simulink model "Demo_AUV_VA"  (R2014a)
settings: Solver=FixedStepDiscrete  StartTime=0.0  StopTime=inf  FixedStep=0.01  RelTol=1e-3
undefined symbols (not defined in the file or in its folder): clock, lib_affectiveChar_behavior, notImitateSmile, Stateflow
libraries: simulink x6, realtime_pacer_lib x2
(part 1 of 2)
settings Model: Creator=root180  LastModifiedBy=root180

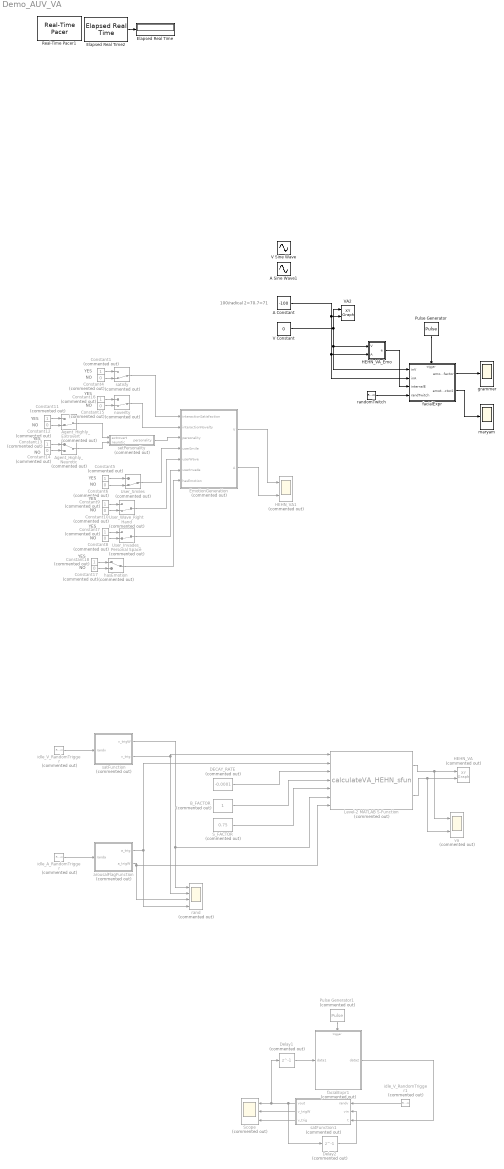
== system Demo_AUV_VA ==
  note: 100/radical 2=70.7=71
  note: NO
  note: NO
  note: YES
  note: YES
  note: NO
  note: YES
  note: NO
  note: NO
  note: NO
  note: NO
  note: NO
  note: YES
  note: YES
  note: YES
  note: YES
  note: YES
  A Constant : Constant  Value=-100
  A Sine Wave1 : Sin  Amplitude=100  Frequency=0.1  SampleTime=0.01
  Agent_Highly_Extrovert : ManualSwitch  Commented=on  CurrentSetting=0
  Agent_Highly_Neurotic : ManualSwitch  Commented=on
  B_FACTOR : Constant  Commented=on
  Constant{1,5,7,9,16,18} (6 alike) : Constant  Commented=on  OutDataTypeStr=double
  Constant{4,6,8,10,15,17} (6 alike) : Constant  Commented=on  Value=0  OutDataTypeStr=double
  Constant11 : Constant  Commented=on  OutDataTypeStr=boolean
  Constant12 : Constant  Commented=on  Value=0  OutDataTypeStr=boolean
  Constant13 : Constant  Commented=on  OutDataTypeStr=boolean
  Constant14 : Constant  Commented=on  Value=0  OutDataTypeStr=boolean
  DECAY_RATE : Constant  Commented=on  Value=-0.0001
  Delay1 : Delay  Commented=on  DelayLength=1  InitialCondition=0  SampleTime=0.01
  Delay2 : Delay  Commented=on  DelayLength=1  InitialCondition=0  SampleTime=0.01
  Elapsed Real Time : Display
      settings: Decimation=2
  Elapsed Real Time2 : realtime_pacer_lib/Elapsed Real Time
  EmotionGeneration : Subsystem  Commented=on
  HEHN_VA : simulink/Sinks/XY Graph  Commented=on  xmin=-110  xmax=100  ymin=-110  ymax=110  st=-1
  HEHN_VA1 : Scope  Commented=on  NumInputPorts=2
      settings: YMin=-0.65~21.8  YMax=0.3~23.9  SaveName=ScopeData4
  HEHN_VA_Emo : Truth Table  TreatAsAtomicUnit=on
  Level-2 MATLAB S-Function : M-S-Function  Commented=on  FunctionName=calculateVA_HEHN_sfun
  Pulse Generator : DiscretePulseGenerator  SampleTime=0.01
  Pulse Generator1 : DiscretePulseGenerator  Commented=on  Period=20  PulseWidth=10  SampleTime=0.01
  Real-Time Pacer1 : realtime_pacer_lib/Real-Time Pacer  simTimePerRealTime=1
  S_FACTOR : Constant  Commented=on  Value=0.75
  Scope : Scope  Commented=on  NumInputPorts=3
      settings: YMin=0.57~0.285~0.95  YMax=0.63~0.315~1.05  SaveName=ScopeData7
  User_Invades_Personal Space : ManualSwitch  Commented=on  CurrentSetting=0
  User_Smiles : ManualSwitch  Commented=on  CurrentSetting=0
  User_Wave_Right Hand : ManualSwitch  Commented=on  CurrentSetting=0
  V Constant : Constant  Value=0
  V Sine Wave : Sin  Amplitude=100  SampleTime=0.01
  VA2 : simulink/Sinks/XY Graph  xmin=-110  xmax=100  ymin=-110  ymax=110  st=-1
  arousalFlagFunction : MATLAB Function  Commented=on  TreatAsAtomicUnit=on
  facialExpr : Stateflow chart  TreatAsAtomicUnit=on
  facialExpr1 : Stateflow chart  Commented=on  TreatAsAtomicUnit=on
  grammer : Scope
  hasEmotion : ManualSwitch  Commented=on
  idle_A_RandomTrigger : UniformRandomNumber  Commented=on  Minimum=0  Maximum=100.9999  Seed=sum(10*clock)  SampleTime=0.1
  idle_V_RandomTrigger : UniformRandomNumber  Commented=on  Minimum=0  Maximum=100.9999  Seed=sum(10*clock)  SampleTime=0.1
  idle_V_RandomTrigger1 : UniformRandomNumber  Commented=on  Minimum=0  Maximum=100.9999  Seed=sum(10*clock)  SampleTime=0.01
  maryam : Scope
      settings: SaveName=ScopeData8
  noverlty : ManualSwitch  Commented=on  CurrentSetting=0
  rand : Scope  Commented=on  NumInputPorts=4
      settings: TickLabels=on  YMin=0~-1~-90~-5  YMax=1~1~-20~5  SaveName=ScopeData2  MaxDataPoints=100000
  randomTwitch : UniformRandomNumber  Minimum=0  Maximum=100.9999  Seed=sum(10*clock)  SampleTime=0.01
  satFunction : MATLAB Function  Commented=on  TreatAsAtomicUnit=on
  satFunction1 : MATLAB Function  Commented=on  TreatAsAtomicUnit=on
  satisfy : ManualSwitch  Commented=on  CurrentSetting=0
  setPersonality : MATLAB Function  Commented=on  TreatAsAtomicUnit=on
  va : Scope  Commented=on  NumInputPorts=2
      settings: YMin=-5~-5  YMax=5~5  SaveName=ScopeData3
  wires:
  Pulse Generator/1 -> facialExpr/Trigger
  facialExpr/1(emotion_amount_factor) -> grammer/1
  V Constant/1 -> VA2/1, HEHN_VA_Emo/1(V), facialExpr/1(inV)
  A Constant/1 -> facialExpr/2(inA), HEHN_VA_Emo/2(A), VA2/2
  EmotionGeneration/1(V) -> HEHN_VA1/1
  EmotionGeneration/2(A) -> HEHN_VA1/2
  User_Invades_Personal Space/1 -> EmotionGeneration/6(userInvade)
  User_Smiles/1 -> EmotionGeneration/4(userSmile)
  setPersonality/1(personality) -> EmotionGeneration/3(personality)
  hasEmotion/1 -> EmotionGeneration/7(hasEmotion)
  Constant9/1 -> User_Wave_Right Hand/1
  Constant11/1 -> Agent_Highly_Extrovert/1
  Constant13/1 -> Agent_Highly_Neurotic/1
  Constant1/1 -> satisfy/1
  Constant6/1 -> User_Smiles/2
  Constant12/1 -> Agent_Highly_Extrovert/2
  Constant18/1 -> hasEmotion/1
  Constant8/1 -> User_Invades_Personal Space/2
  Agent_Highly_Neurotic/1 -> setPersonality/2(neurotic)
  Constant15/1 -> noverlty/2
  Constant17/1 -> hasEmotion/2
  Constant7/1 -> User_Invades_Personal Space/1
  Constant4/1 -> satisfy/2
  Constant10/1 -> User_Wave_Right Hand/2
  noverlty/1 -> EmotionGeneration/2(interactionNovelty)
  Constant16/1 -> noverlty/1
  Constant5/1 -> User_Smiles/1
  User_Wave_Right Hand/1 -> EmotionGeneration/5(userWave)
  Agent_Highly_Extrovert/1 -> setPersonality/1(extrovert)
  satisfy/1 -> EmotionGeneration/1(interactionSatisfaction)
  Constant14/1 -> Agent_Highly_Neurotic/2
  idle_V_RandomTrigger/1 -> satFunction/1(randv)
  B_FACTOR/1 -> Level-2 MATLAB S-Function/4
  DECAY_RATE/1 -> Level-2 MATLAB S-Function/3
  idle_A_RandomTrigger/1 -> arousalFlagFunction/1(randa)
  S_FACTOR/1 -> Level-2 MATLAB S-Function/5
  Level-2 MATLAB S-Function/2 -> va/2, HEHN_VA/2
  Level-2 MATLAB S-Function/1 -> va/1, HEHN_VA/1
  satFunction/2(v_trig) -> rand/2, Level-2 MATLAB S-Function/1
  arousalFlagFunction/1(a_trig) -> rand/4, Level-2 MATLAB S-Function/2
  arousalFlagFunction/2(a_trigW) -> Level-2 MATLAB S-Function/7, rand/3
  satFunction/1(v_trigW) -> Level-2 MATLAB S-Function/6, rand/1
  Elapsed Real Time2/1 -> Elapsed Real Time/1
  idle_V_RandomTrigger1/1 -> satFunction1/1(randv)
  satFunction1/1(vout) -> Delay2/1, Scope/1, Delay1/1
  satFunction1/3(v_trig) -> Scope/3
  satFunction1/2(v_trigW) -> Scope/2
  Pulse Generator1/1 -> facialExpr1/Trigger
  Delay1/1 -> facialExpr1/1(data1)
  facialExpr1/1(data2) -> satFunction1/3(t)
  Delay2/1 -> satFunction1/2(vin)
  HEHN_VA_Emo/1(e) -> facialExpr/3(internalE)
  facialExpr/2(emotion_amount_factor2) -> maryam/1
  randomTwitch/1 -> facialExpr/4(randTwitch)

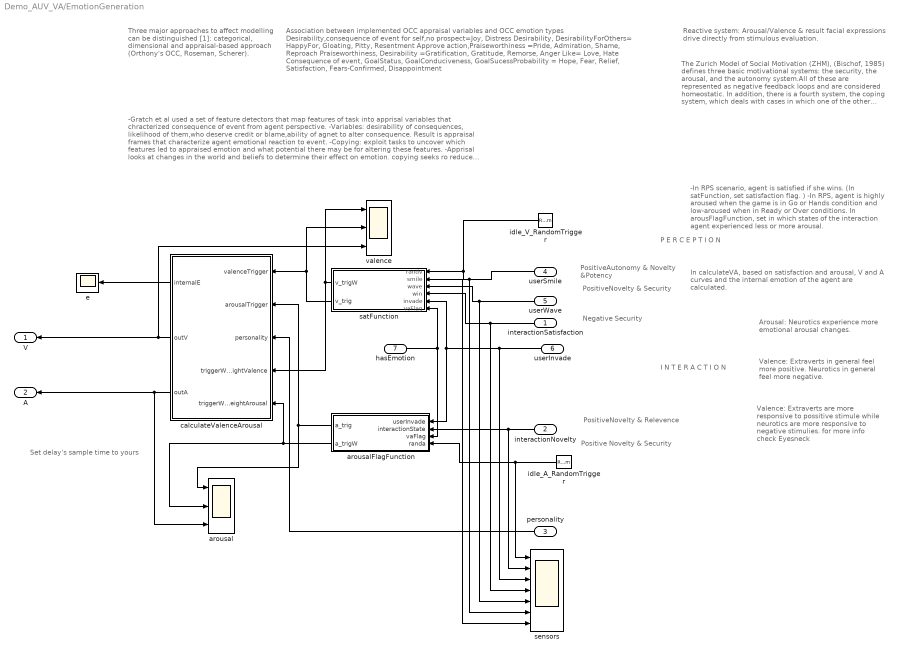
== system Demo_AUV_VA/EmotionGeneration ==
  note: P
      | E
      | R
      | C
      | E
      | P
      | T
      | I
      | O
      | N
  note: PositiveNovelty &
      | Relevence
  note: The Zurich Model of Social Motivation (ZHM), (Bischof, 1985) defines three basic motivational systems: the security, the arousal, and the autonomy system.All of these are represented as negative feedback loops and are considered homeostatic. In addition, there is a fourth system, the coping system, which deals with cases in which one of the other systems gets blocked and cannot operate in its usual manner.( Bernardet and Schneider, 2013)
  note: PositiveNovelty &
      | Security
  note: Three major approaches to affect modelling can be distinguished [1]: categorical, dimensional and appraisal-based approach (Orthony's OCC, Roseman, Scherer).
  note: Reactive system: Arousal/Valence & result facial expressions drive directly from stimulous evaluation.
  note: Association between implemented OCC appraisal variables and OCC emotion types
      | Desirability,consequence of event for self,no prospect=Joy, Distress
      | Desirability, DesirabilityForOthers= HappyFor, Gloating, Pitty, Resentment
      | Approve action,Praiseworthiness =Pride, Admiration, Shame, Reproach
      | Praiseworthiness, Desirability =Gratification, Gratitude, Remorse, Anger
      | Like= Love, Hate
      | Consequence of event, GoalStatus, GoalConduciveness, GoalSucessProbability = Hope, Fear, Relief, Satisfaction, Fears-Confirmed, Disappointment
  note: -Gratch et al used a set of feature detectors that map features of task into apprisal variables that chracterized consequence of event from agent perspective.
      | -Variables: desirability of consequences, likelihood of them,who deserve credit or blame,ability of agnet to alter consequence. Result is appraisal frames that characterize agent emotional reaction to event.
      | -Copying: exploit tasks to uncover which features led to appraised emotion and what potential there may be for altering these features.
      | -Apprisal looks at changes in the world and beliefs to determine their effect on emotion.
      | copying seeks ro reduce (-) emotions by making changes to world or beliefs (problem-focused v.s. emotion-focused)
      | -For more info check Toward Virtual Humans, Swartout,w., et al (2006)
  note: In calculateVA, based on satisfaction and arousal, V and A curves and the internal emotion of the agent are calculated.
  note: Set delay's sample time to yours
  note: -In RPS scenario, agent is satisfied if she wins. (In satFunction, set satisfaction flag. )
      | -In RPS, agent is highly aroused when the game is in Go or Hands condition and low-aroused when in Ready or Over conditions.
      | In arousFlagFunction, set in which states of the interaction agent experienced less or more arousal.
  note: Valence: Extraverts are more responsive to possitive stimule while neurotics are more responsive to negative stimulies. for more info check Eyesneck
  note: Valence: Extraverts in general feel more positive. Neurotics in general feel more negative.
  note: Arousal: Neurotics experience more emotional arousal changes.
  note: Positive Novelty &
      | Security
  note: Negative Security
  note: PositiveAutonomy &
      | Novelty &Potency
  note: I
      | N
      | T
      | E
      | R
      | A
      | C
      | T
      | I
      | O
      | N
  interactionSatisfaction : Inport
  interactionNovelty : Inport  Port=2
  personality : Inport  Port=3
  userSmile : Inport  Port=4
  userWave : Inport  Port=5
  userInvade : Inport  Port=6
  hasEmotion : Inport  Port=7
  arousal : Scope  NumInputPorts=3
      settings: TickLabels=on  YMin=-1~0~0  YMax=1~0.1~90  SaveName=ScopeData12  MaxDataPoints=200000
  arousalFlagFunction : MATLAB Function  TreatAsAtomicUnit=on
  calculateValenceArousal : Subsystem
  e : Scope
      settings: TickLabels=on  YMin=0  YMax=1  MaxDataPoints=100000
  idle_A_RandomTrigger : UniformRandomNumber  Minimum=0  Maximum=100.9999  Seed=sum(10*clock)  SampleTime=0.01
  idle_V_RandomTrigger : UniformRandomNumber  Minimum=0  Maximum=100.9999  Seed=sum(10*clock)  SampleTime=0.01
  satFunction : MATLAB Function  TreatAsAtomicUnit=on
  sensors : Scope  NumInputPorts=7
      settings: YMin=0.95~-20.15~-20.15~-5~-5~-5~-5  YMax=1.05~-19.15~-19.15~5~5~5~5  SaveName=ScopeData10  MaxDataPoints=20000
  valence : Scope  NumInputPorts=3
      settings: TickLabels=on  YMin=0~-1~-90  YMax=1~1~-20  SaveName=ScopeData14  MaxDataPoints=100000
  V : Outport
  A : Outport  Port=2
  wires:
  arousalFlagFunction/1(a_trig) -> calculateValenceArousal/2(arousalTrigger), arousal/1
  calculateValenceArousal/2(outV) -> V/1, valence/3
  calculateValenceArousal/3(outA) -> A/1, arousal/3
  personality/1 -> calculateValenceArousal/3(personality)
  interactionNovelty/1 -> sensors/2, arousalFlagFunction/2(interactionState)
  interactionSatisfaction/1 -> sensors/4, satFunction/4(win)
  userInvade/1 -> sensors/3, arousalFlagFunction/1(userInvade), satFunction/5(invade)
  userWave/1 -> sensors/5, satFunction/3(wave)
  satFunction/1(v_trigW) -> valence/1, calculateValenceArousal/4(triggerWeightValence)
  arousalFlagFunction/2(a_trigW) -> arousal/2, calculateValenceArousal/5(triggerWeightArousal)
  hasEmotion/1 -> satFunction/6(vaFlag), arousalFlagFunction/3(vaFlag)
  idle_V_RandomTrigger/1 -> sensors/7, satFunction/1(randv)
  idle_A_RandomTrigger/1 -> sensors/1, arousalFlagFunction/4(randa)
  satFunction/2(v_trig) -> calculateValenceArousal/1(valenceTrigger), valence/2
  calculateValenceArousal/1(internalE) -> e/1
  userSmile/1 -> satFunction/2(smile), sensors/6

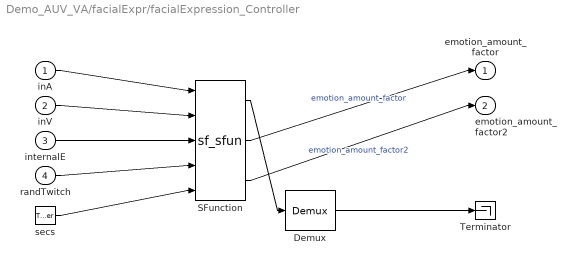
== system Demo_AUV_VA/facialExpr/facialExpression_Controller ==
  inA : Inport
  inV : Inport  Port=2
  internalE : Inport  Port=3
  randTwitch : Inport  Port=4
  secs : TriggerPort  ShowOutputPort=on
  " Demux " : Demux  Outputs=1
  " SFunction " : S-Function  Tag=Stateflow S-Function Demo_AUV_VA 50  FunctionName=sf_sfun  PortCounts=[5 3]  EnableBusSupport=off
  " Terminator " : Terminator
  emotion_amount_factor : Outport
  emotion_amount_factor2 : Outport  Port=2
  wires:
  inA/1 -> " SFunction "/1
  inV/1 -> " SFunction "/2
  internalE/1 -> " SFunction "/3
  randTwitch/1 -> " SFunction "/4
  " SFunction "/2 -> emotion_amount_factor/1  "emotion_amount_factor"
  " SFunction "/3 -> emotion_amount_factor2/1  "emotion_amount_factor2"
  " Demux "/1 -> " Terminator "/1
  secs/1 -> " SFunction "/5
  " SFunction "/1 -> " Demux "/1

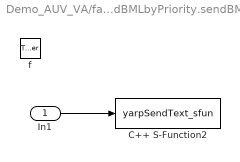
== system Demo_AUV_VA/facialExpr/sendBMLbyPriority.sendBML ==
  In1 : Inport  OutDataTypeStr=double  PortDimensions=[2000 1]
  f : TriggerPort  TriggerType=function-call
      settings: CopyFcn=Stateflow.SLINSF.SimulinkMan.removeBlockPreDeleteFcn  PreDeleteFcn=Stateflow.SLINSF.SimulinkMan.unsafePredeleteFcn
  C++ S-Function2 : S-Function  FunctionName=yarpSendText_sfun  Parameters='/sim/out/bml0', '/SB/in/bml'  EnableBusSupport=off
  wires:
  In1/1 -> C++ S-Function2/1

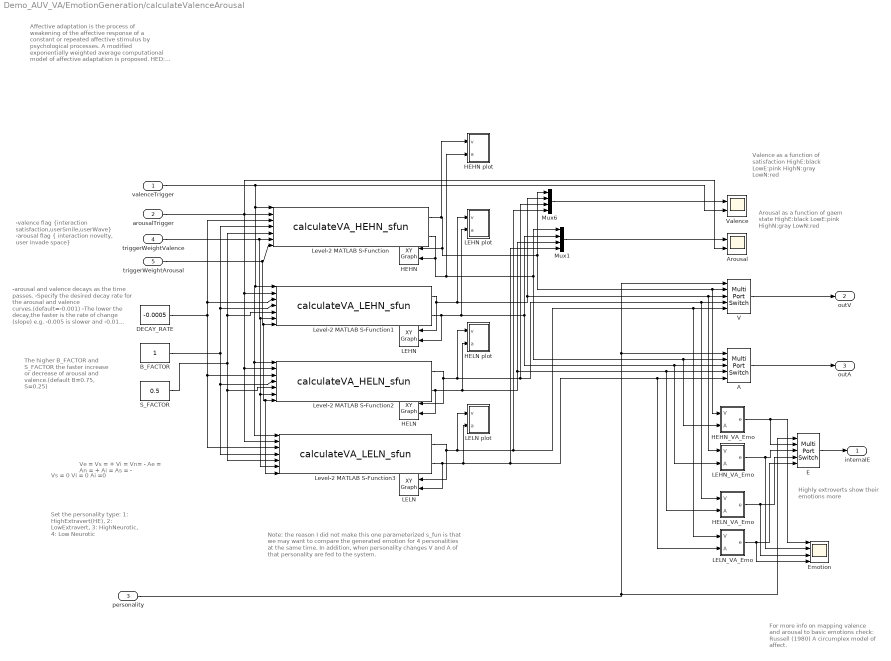
== system Demo_AUV_VA/EmotionGeneration/calculateValenceArousal ==
  note: Highly extroverts show their emotions more
  note: Note: the reason I did not make this one parameterized s_fun is that we may want to compare the generated emotion for 4 personalities at the same time.
      | In addition, when personality changes V and A of that personality are fed to the system.
  note: For more info on mapping valence and arousal to basic emotions check: Russell (1980) A circumplex model of affect.
  note: Valence as a  function of satisfaction
      | HighE:black
      | LowE:pink
      | HighN:gray
      | LowN:red
  note: Set the personality type:
      | 1: HighExtravert(HE),
      | 2: LowExtravert,
      | 3: HighNeurotic,
      | 4: Low Neurotic
  note: The higher B_FACTOR and S_FACTOR the faster increase or decrease of arousal and valence.(default B=0.75, S=0.25)
  note: -arousal and valence decays as the time passes.
      | -Specify the desired decay rate for the arousal and valence curves.(default=-0.001)
      | -The lower the decay,the faster is the rate of change (slope)
      | e.g. -0.005 is slower and -0.01 faster
  note: Vs = 0
      | Vi = 0
      | Ai =0
  note: Ve = Vs = +
      | Vi = Vn= -
      | Ae = An = +
      | Ai = As  = -
  note: Arousal as a function of gaem state
      | HighE:black
      | LowE:pink
      | HighN:gray
      | LowN:red
  note: Affective adaptation is the process of weakening of the affective response of a constant or repeated affective stimulus by psychological processes. A modified exponentially weighted average computational model of affective adaptation is proposed.
      |
      | HED: A Computational Model of Affective Adaptation and Emotion Dynamics, John E. Steephen
  note: -valence flag {interaction satisfaction,userSmile,userWave}
      | -arousal flag { interaction novelty, user invade space}
  valenceTrigger : Inport  OutDataTypeStr=double  PortDimensions=1
  arousalTrigger : Inport  Port=2  OutDataTypeStr=double  PortDimensions=1
  personality : Inport  Port=3  OutDataTypeStr=double  PortDimensions=1
  triggerWeightValence : Inport  Port=4  OutDataTypeStr=double  PortDimensions=1
  triggerWeightArousal : Inport  Port=5  OutDataTypeStr=double  PortDimensions=1
  A : MultiPortSwitch  Inputs=4
  Arousal : Scope  NumInputPorts=2
      settings: YMin=-6~-1  YMax=5~1  SaveName=ScopeData11  MaxDataPoints=20000
  B_FACTOR : Constant
  DECAY_RATE : Constant  Value=-0.0005
  E : MultiPortSwitch  Inputs=4
  Emotion : Scope  NumInputPorts=4
      settings: TimeRange=50  YMin=6.65~5.7~5.7~5.7  YMax=7.35~6.3~6.3~6.3  SaveName=ScopeData5  MaxDataPoints=10000
  HEHN : simulink/Sinks/XY Graph  xmin=-110  xmax=100  ymin=-110  ymax=110  st=-1
  HEHN plot : MATLAB Function  TreatAsAtomicUnit=on
  HEHN_VA_Emo : Truth Table  TreatAsAtomicUnit=on
  HELN : simulink/Sinks/XY Graph  xmin=-110  xmax=110  ymin=-110  ymax=110  st=-1
  HELN plot : MATLAB Function  TreatAsAtomicUnit=on
  HELN_VA_Emo : Truth Table  TreatAsAtomicUnit=on
  LEHN : simulink/Sinks/XY Graph  xmin=-110  xmax=110  ymin=-110  ymax=110  st=-1
  LEHN plot : MATLAB Function  TreatAsAtomicUnit=on
  LEHN_VA_Emo : Truth Table  TreatAsAtomicUnit=on
  LELN : simulink/Sinks/XY Graph  xmin=-110  xmax=110  ymin=-110  ymax=110  st=-1
  LELN plot : MATLAB Function  TreatAsAtomicUnit=on
  LELN_VA_Emo : Truth Table  TreatAsAtomicUnit=on
  Level-2 MATLAB S-Function : M-S-Function  FunctionName=calculateVA_HEHN_sfun
  Level-2 MATLAB S-Function1 : M-S-Function  FunctionName=calculateVA_LEHN_sfun
  Level-2 MATLAB S-Function2 : M-S-Function  FunctionName=calculateVA_HELN_sfun
  Level-2 MATLAB S-Function3 : M-S-Function  FunctionName=calculateVA_LELN_sfun
  Mux1 : Mux
  Mux6 : Mux
  S_FACTOR : Constant  Value=0.5
  V : MultiPortSwitch  Inputs=4
  Valence : Scope  NumInputPorts=2
      settings: TimeRange=10  YMin=-12~-1  YMax=10~1  SaveName=ScopeData6  MaxDataPoints=20000
  internalE : Outport
  outV : Outport  Port=2
  outA : Outport  Port=3
  wires:
  valenceTrigger/1 -> Valence/2, Level-2 MATLAB S-Function/1, Level-2 MATLAB S-Function3/1, Level-2 MATLAB S-Function2/1, Level-2 MATLAB S-Function1/1
  Level-2 MATLAB S-Function/2 -> HEHN/2, HEHN plot/2(a), HEHN_VA_Emo/2(A), A/2, Mux1/1
  arousalTrigger/1 -> Arousal/2, Level-2 MATLAB S-Function/2, Level-2 MATLAB S-Function3/2, Level-2 MATLAB S-Function2/2, Level-2 MATLAB S-Function1/2
  Level-2 MATLAB S-Function1/2 -> LEHN plot/2(a), LEHN_VA_Emo/2(A), A/3, Mux1/2, LEHN/2
  Level-2 MATLAB S-Function/1 -> HEHN plot/1(v), Mux6/1, HEHN_VA_Emo/1(V), V/2, HEHN/1
  Level-2 MATLAB S-Function1/1 -> LEHN plot/1(v), Mux6/2, LEHN_VA_Emo/1(V), V/3, LEHN/1
  Level-2 MATLAB S-Function2/2 -> HELN plot/2(a), Mux1/3, HELN_VA_Emo/2(A), A/4, HELN/2
  Level-2 MATLAB S-Function3/2 -> LELN plot/2(a), LELN_VA_Emo/2(A), A/5, Mux1/4, LELN/2
  Level-2 MATLAB S-Function2/1 -> HELN plot/1(v), HELN_VA_Emo/1(V), V/4, Mux6/3, HELN/1
  Level-2 MATLAB S-Function3/1 -> LELN plot/1(v), LELN_VA_Emo/1(V), V/5, Mux6/4, LELN/1
  Mux1/1 -> Arousal/1
  Mux6/1 -> Valence/1
  DECAY_RATE/1 -> Level-2 MATLAB S-Function/3, Level-2 MATLAB S-Function1/3, Level-2 MATLAB S-Function2/3, Level-2 MATLAB S-Function3/3
  B_FACTOR/1 -> Level-2 MATLAB S-Function/4, Level-2 MATLAB S-Function1/4, Level-2 MATLAB S-Function3/4, Level-2 MATLAB S-Function2/4
  S_FACTOR/1 -> Level-2 MATLAB S-Function3/5, Level-2 MATLAB S-Function2/5, Level-2 MATLAB S-Function1/5, Level-2 MATLAB S-Function/5
  V/1 -> outV/1
  A/1 -> outA/1
  personality/1 -> E/1, V/1, A/1
  triggerWeightValence/1 -> Level-2 MATLAB S-Function3/6, Level-2 MATLAB S-Function2/6, Level-2 MATLAB S-Function1/6, Level-2 MATLAB S-Function/6
  triggerWeightArousal/1 -> Level-2 MATLAB S-Function3/7, Level-2 MATLAB S-Function2/7, Level-2 MATLAB S-Function1/7, Level-2 MATLAB S-Function/7
  HEHN_VA_Emo/1(e) -> Emotion/1, E/2
  LEHN_VA_Emo/1(e) -> Emotion/2, E/3
  HELN_VA_Emo/1(e) -> Emotion/3, E/4
  LELN_VA_Emo/1(e) -> Emotion/4, E/5
  E/1 -> internalE/1

== matlab function Demo_AUV_VA/arousalFlagFunction ==
  data: a_trig output; a_trigW output; randa input
function [a_trig,a_trigW]= fcn(randa)
    a_trigW=0; 
    randTrigger=floor(randa);
    if(0<randTrigger)&&(randTrigger<30)
        a_trigW = a_trigW + 0.3;
    end
    if(30<randTrigger)&&(randTrigger<60)
        a_trigW = a_trigW - 0.3;
    end

    if(a_trigW>0)
        a_trig=1;
    elseif(a_trigW<0)
        a_trig=-1;
        a_trigW=abs(a_trigW);
    else
        a_trig=0;
    end

== matlab function Demo_AUV_VA/satFunction ==
  data: randv input; v_trigW output; v_trig output
function [v_trigW,v_trig]= fcn(randv)
    
    v_trigW=0;
    
    randTrigger=floor(randv);
    
    if(0<randTrigger)&&(randTrigger<30)
        v_trigW = v_trigW + 0.3;
    end
    if(30<randTrigger)&&(randTrigger<60)
        v_trigW = v_trigW - 0.3;
    end

    if(v_trigW>0)
        v_trig=1;
    elseif(v_trigW<0)
        v_trig=-1;
        v_trigW=abs(v_trigW);
    else
        v_trig=0;v_trigW=0;
    end

== stateflow chart Demo_AUV_VA/facialExpr ==
  state facialExpression_Controller [parallel]
    settings: executionOrder=1
  state sendBMLbyPriority [parallel]
    settings: executionOrder=2
    state sendH
      entry: BML=bmlsH(:,1);
      sendBML(BML);
      newBmlsH=removeQueue(bmlsH);
      bmlsH=newBmlsH;
    state init
      entry: n=encStr2Arr(' ');
      bmlsH=[n n n n n];
      bmlsM=[n n n n n];
      bmlsL=[n n n n n];
    state checkHighPriority
      entry:
      hEmpty=isEmptyQueue(bmlsH);
    state sendM
      entry: BML=bmlsM(:,1);
      sendBML(BML);
      newBmlsM= removeQueue(bmlsM);
      bmlsM=newBmlsM;
    state Mid
      entry:mEmpty=isEmptyQueue(bmlsM);
    state sendL
      entry: BML=bmlsL(:,1);
      sendBML(BML);
      newBmlsL= removeQueue(bmlsL);
      bmlsL=newBmlsL;
    state low
      entry:
      lEmpty=isEmptyQueue(bmlsL);
    note: Arrows' execution order is very importan here!
    state sendBML(In1) [function]
    sendH -> checkHighPriority
    checkHighPriority -> sendH [order 2] : [hEmpty~=1]
    (default) -> init
    init -> checkHighPriority
    checkHighPriority -> Mid [order 1] : [hEmpty==1]
    Mid -> checkHighPriority [order 4] : [mEmpty==1]
    sendM -> checkHighPriority [order 2]
    sendL -> checkHighPriority [order 3]
    low -> sendH [order 1] : [isEmptyQueue(bmlsH)~=1]
    Mid -> sendH [order 1] : [isEmptyQueue(bmlsH)~=1]
    sendM -> sendH [order 1] : [isEmptyQueue(bmlsH)~=1]
    sendL -> sendH [order 2] : [isEmptyQueue(bmlsH)~=1]
    Mid -> sendM [order 2] : [mEmpty~=1]
    Mid -> low [order 3] : [mEmpty==1]
    low -> Mid [order 4] : [lEmpty==1]
    low -> sendM [order 2] : [isEmptyQueue(bmlsM)~=1]
    sendL -> sendM [order 1] : [isEmptyQueue(bmlsM)~=1]
    low -> sendL [order 3] : [lEmpty~=1]
  data: In1 function_input double size=[2000 1]; bmls function_input; newBmls function_output; bmls function_input; empty function_output; inV input double size=1; inA input double size=1; bmlsL local double size=[2000,5]; newBmlsL local double size=[2000,5]; emotion_amount_factor output double size=[1,15]; hEmpty local double size=1; newBmlsM local double size=[2000,5]; bmlsM local double size=[2000,5]; newBmlsH local double size=[2000,5]; bmlsH local double size=[2000,5]; newBmlA local; BML local double size=[2000,1]; lEmpty local; mEmpty local; n local double size=[2000,1]; internalE input double size=1; emotion_amount_factor2 output double size=[1,6]; randTwitch input double size=1
  events: secs input RISING_EDGE_EVENT
  function newBmls=removeQueue(bmls):
    | function newBmls=removeQueue(bmls) 
    |     n=encStr2Arr(' ');
    |     newBmls=[n n n n n];
    |     newBmls(:,1)= bmls(:,2);
    |     newBmls(:,2)= bmls(:,3);
    |     newBmls(:,3)= bmls(:,4);
    |     newBmls(:,4)= bmls(:,5);
    |     newBmls(:,5)=encStr2Arr(' ');
  function empty=isEmptyQueue(bmls):
    | function empty=isEmptyQueue(bmls)
    | empty=1;
    | tempp=encStr2Arr(' ');
    | for i = 1:5
    |     if (isequal(bmls(:,i),tempp)==0)%there is a cell which is not equal to null
    |         empty=0;
    |         break
    |     end
    | end

== matlab function Demo_AUV_VA/satFunction1 ==
  data: vout output; randv input; v_trigW output; v_trig output; vin input; t input
function [vout,v_trigW,v_trig]= fcn(randv,vin,t)
%#codegen
    v_trigW=0;vout=0;
    randTrigger=floor(randv);
    if(0<randTrigger)&&(randTrigger<30)
        v_trigW = v_trigW + 0.3;
    end
    if(30<randTrigger)&&(randTrigger<60)
        v_trigW = v_trigW - 0.3;
    end
    if(v_trigW>0)
        v_trig=1;
    elseif(v_trigW<0)
        v_trig=-1;
        v_trigW=abs(v_trigW);
    else
        v_trig=0;
    end
    
    if v_trig==1           
            vout = vin + (1*v_trigW); %V=s-/i-s/d-f 
    end
    if v_trig== -1 %HEHN highly responsive to negative stimuli
            vout =vin - (1*v_trigW);  
                %rate = -0.01;
    end

== matlab function Demo_AUV_VA/HEHN_VA_Emo ==
  data: V input; e output double size=1; A input double
function e = fcn(V, A)

aVarTruthTableCondition_1 = false;
aVarTruthTableCondition_2 = false;
aVarTruthTableCondition_3 = false;
aVarTruthTableCondition_4 = false;
aVarTruthTableCondition_5 = false;
aVarTruthTableCondition_6 = false;
aVarTruthTableCondition_7 = false;
aVarTruthTableCondition_8 = false;


% 7-happy  2,1

aVarTruthTableCondition_1 = logical(V>10 && A<40 && A>10);

% 8-ex  1,2 AND 2,2

aVarTruthTableCondition_2 = logical(V>0 && A>40);

% 4-fear  -1,2 AND -2,2

aVarTruthTableCondition_3 = logical(V<0 && A>40);

% 3-frust  -2,1

aVarTruthTableCondition_4 = logical(V<-10 && A<40 && A>10);

% 6-pleased  2,-1

aVarTruthTableCondition_5 = logical(V>10 && A<-10 && A>-40);

% 5-calm  1,-2 AND 2,-2

aVarTruthTableCondition_6 = logical(V>0 && A<-40);

% 1-bored  -1,-2 AND -2,-2

aVarTruthTableCondition_7 = logical(V<0 && A<-40);

% 2-sad  -2,-1

aVarTruthTableCondition_8 = logical(V<-10 && A<-10 && A>-40);

if (aVarTruthTableCondition_1)
    aFcnTruthTableAction_1();
elseif (aVarTruthTableCondition_2)
    aFcnTruthTableAction_2();
elseif (aVarTruthTableCondition_3)
    aFcnTruthTableAction_3();
elseif (aVarTruthTableCondition_4)
    aFcnTruthTableAction_4();
elseif (aVarTruthTableCondition_5)
    aFcnTruthTableAction_5();
elseif (aVarTruthTableCondition_6)
    aFcnTruthTableAction_6();
elseif (aVarTruthTableCondition_7)
    aFcnTruthTableAction_7();
elseif (aVarTruthTableCondition_8)
    aFcnTruthTableAction_8();
else % Default
    aFcnTruthTableAction_5();
end

function aFcnTruthTableAction_1()

% happy

e=7;

function aFcnTruthTableAction_2()

% excited

e=8;

function aFcnTruthTableAction_3()

% fear

e=4;

function aFcnTruthTableAction_4()

% frustration

e=3;

function aFcnTruthTableAction_5()

% pleased

e=6;

function aFcnTruthTableAction_6()

% contempt

e=5;

function aFcnTruthTableAction_7()

% bored

e=1;

function aFcnTruthTableAction_8()

% sad

e=2;

== stateflow chart Demo_AUV_VA/facialExpr1 ==
  state s
    entry:
  state s2
    entry: data2=data1;
  (default) -> s
  s -> s2 : after(20,secs)
  data: data1 input double size=1; data2 output double size=1
  events: secs input RISING_EDGE_EVENT

== matlab function Demo_AUV_VA/EmotionGeneration/calculateValenceArousal/LEHN_VA_Emo ==
  data: V input; e output double size=1; A input double
function e = fcn(V, A)

aVarTruthTableCondition_1 = false;
aVarTruthTableCondition_2 = false;
aVarTruthTableCondition_3 = false;
aVarTruthTableCondition_4 = false;
aVarTruthTableCondition_5 = false;
aVarTruthTableCondition_6 = false;
aVarTruthTableCondition_7 = false;
aVarTruthTableCondition_8 = false;


% 7-happy  2,1

aVarTruthTableCondition_1 = logical(V>20 && A<40 && A>20);

% 8-ex  1,2 AND 2,2

aVarTruthTableCondition_2 = logical(V>0 && A>40);

% 4-fear  -1,2 AND -2,2

aVarTruthTableCondition_3 = logical(V<0 && A>40);

% 3-frust  -2,1

aVarTruthTableCondition_4 = logical(V<-20 && A<40 && A>20);

% 6-idle  2,-1

aVarTruthTableCondition_5 = logical(V>20 && A<-20 && A>-40);

% 5-calm  1,-2 AND 2,-2

aVarTruthTableCondition_6 = logical(V>0 && A<-40);

% 1-bored  -1,-2 AND -2,-2

aVarTruthTableCondition_7 = logical(V<0 && A<-40);

% 2-sad  -2,-1

aVarTruthTableCondition_8 = logical(V<-20 && A<-20 && A>-40);

if (aVarTruthTableCondition_1)
    aFcnTruthTableAction_1();
elseif (aVarTruthTableCondition_2)
    aFcnTruthTableAction_2();
elseif (aVarTruthTableCondition_3)
    aFcnTruthTableAction_3();
elseif (aVarTruthTableCondition_4)
    aFcnTruthTableAction_4();
elseif (aVarTruthTableCondition_5)
    aFcnTruthTableAction_5();
elseif (aVarTruthTableCondition_6)
    aFcnTruthTableAction_6();
elseif (aVarTruthTableCondition_7)
    aFcnTruthTableAction_7();
elseif (aVarTruthTableCondition_8)
    aFcnTruthTableAction_8();
else % Default
    aFcnTruthTableAction_5();
end

function aFcnTruthTableAction_1()

% happy

e=7;

function aFcnTruthTableAction_2()

% excited

e=8;

function aFcnTruthTableAction_3()

% fear

e=4;

function aFcnTruthTableAction_4()

% frustration

e=3;

function aFcnTruthTableAction_5()

% idle

e=6;

function aFcnTruthTableAction_6()

% contempt

e=5;

function aFcnTruthTableAction_7()

% bored

e=1;

function aFcnTruthTableAction_8()

% sad

e=2;

== matlab function Demo_AUV_VA/EmotionGeneration/satFunction ==
  data: randv input; smile input; wave input; win input; invade input; v_trigW output; vaFlag input; v_trig output
function [v_trigW,v_trig]= fcn(randv,smile,wave,win,invade,vaFlag)
%#codegen
% 30/06/2015
    %Here set Agent's satisfaction flag based on your scenario
    %In RPS scenario agent gets satisfined when she wins. states of interaction= {STATE_READY=7;
    %STATE_GO=1;STATE_HAND=2;STATE_OVER=3; STATE_BEFORE=4;STATE_RESULT=5;STATE_WAIT=6;}
   
    if(vaFlag==1)
        v_trigW=0;%weight by which valence value is changed (sum of weight of all triggers)
        %randv 30% chance of random increase or decrease in valence
        randTrigger=floor(randv);
        if(0<randTrigger)&&(randTrigger<30)
            v_trigW = v_trigW + 0.05; %fprintf('v-randp: %0.3f\r\n',v_trigW);
        end
        if(30<randTrigger)&&(randTrigger<60)
            v_trigW = v_trigW - 0.05; %fprintf('v-randn: %0.3f\r\n',v_trigW);
        end

        if(win==2) %agent wins so she is satisfied
            v_trigW = v_trigW + 0.5;
        elseif(win==1) %user wins so agent is NOT satisfied
            v_trigW = v_trigW - 0.5;
        end

        if(smile==1)
            v_trigW=v_trigW+0.25;
        end

        if(wave==1)
            v_trigW=v_trigW+0.25;
        end

        if(invade==1)
            v_trigW=v_trigW-0.25;
        end
    else
         v_trigW=0;
    end
%     fprintf('t: %0.3f\r\n',v_trigW);
    if(v_trigW>0)
        v_trig=1;
    elseif(v_trigW<0)
        v_trig=-1;
        v_trigW=abs(v_trigW);
    else
        v_trig=0;
    end

== matlab function Demo_AUV_VA/EmotionGeneration/arousalFlagFunction ==
  data: userInvade input; interactionState input; a_trig output; a_trigW output; vaFlag input; randa input
function [a_trig,a_trigW]= fcn(userInvade,interactionState,vaFlag,randa)
%#codegen
% 30/06/2015
    %Here set in which states of the interaction agent experienced 
    % more arousal(arousalFlag=1) and less arousal (arousalFlag=-1)
    %Note that you should define the states in your scenraio beforehand
    %we assume agent gets more aroused when in ready/go state and 
    %less aroused when in WAITE/HAND
    if(vaFlag==1)
        a_trigW=0; %weight by which arousal value is changed (sum of weight of all triggers)

        %randa 30% chance of random increase or decrease in arousal
        randTrigger=floor(randa);
        if(0<randTrigger)&&(randTrigger<30)
            a_trigW=a_trigW+0.05;
        end
        if(30<randTrigger)&&(randTrigger<60)
            a_trigW=a_trigW - 0.05;
        end

        if(interactionState==1)%GO - highely aroused state
            a_trigW=a_trigW+0.5;
        end
        if(interactionState==7)%READY - high aroused state
            a_trigW=a_trigW+0.5;
        end
        if(interactionState==2)%HAND- highely aroused state
            a_trigW=a_trigW -0.5;
        end
        if(interactionState==6)%WAIT - low aroused state
            a_trigW=a_trigW-0.5;
        end
        %     elseif(interactionState==3)%OVER - low aroused state
    %         arousalTrig=-1;  
    %         end
        if(userInvade==1)
           a_trigW=a_trigW+0.25;
        end   
    else
        a_trigW=0;
    end
    
    
    if(a_trigW>0)
        a_trig=1;
    elseif(a_trigW<0)
        a_trig=-1;
        a_trigW=abs(a_trigW);
    else
        a_trig=0;
    end

== matlab function Demo_AUV_VA/setPersonality ==
  data: extrovert input; personality output; neurotic input
function personality = fcn(extrovert,neurotic)
%#codegen
% 1 HEHN 2 LEHN 3 HELN 4 LELN
if(extrovert==1)
    if(neurotic==1)
        personality = 1;% 1 HEHN
    else 
        personality = 3;%HELN
    end
else
    if(neurotic==1)
        personality = 2;%LEHN
    else
        personality = 4;%LELN
    end
end

== matlab function Demo_AUV_VA/EmotionGeneration/calculateValenceArousal/HEHN_VA_Emo ==
  data: V input; e output double size=1; A input double
function e = fcn(V, A)

aVarTruthTableCondition_1 = false;
aVarTruthTableCondition_2 = false;
aVarTruthTableCondition_3 = false;
aVarTruthTableCondition_4 = false;
aVarTruthTableCondition_5 = false;
aVarTruthTableCondition_6 = false;
aVarTruthTableCondition_7 = false;
aVarTruthTableCondition_8 = false;


% 7-happy  2,1

aVarTruthTableCondition_1 = logical(V>10 && A<40 && A>10);

% 8-ex  1,2 AND 2,2

aVarTruthTableCondition_2 = logical(V>0 && A>40);

% 4-fear  -1,2 AND -2,2

aVarTruthTableCondition_3 = logical(V<0 && A>40);

% 3-frust  -2,1

aVarTruthTableCondition_4 = logical(V<-10 && A<40 && A>10);

% 6-pleased  2,-1

aVarTruthTableCondition_5 = logical(V>10 && A<-10 && A>-40);

% 5-calm  1,-2 AND 2,-2

aVarTruthTableCondition_6 = logical(V>0 && A<-40);

% 1-bored  -1,-2 AND -2,-2

aVarTruthTableCondition_7 = logical(V<0 && A<-40);

% 2-sad  -2,-1

aVarTruthTableCondition_8 = logical(V<-10 && A<-10 && A>-40);

if (aVarTruthTableCondition_1)
    aFcnTruthTableAction_1();
elseif (aVarTruthTableCondition_2)
    aFcnTruthTableAction_2();
elseif (aVarTruthTableCondition_3)
    aFcnTruthTableAction_3();
elseif (aVarTruthTableCondition_4)
    aFcnTruthTableAction_4();
elseif (aVarTruthTableCondition_5)
    aFcnTruthTableAction_5();
elseif (aVarTruthTableCondition_6)
    aFcnTruthTableAction_6();
elseif (aVarTruthTableCondition_7)
    aFcnTruthTableAction_7();
elseif (aVarTruthTableCondition_8)
    aFcnTruthTableAction_8();
else % Default
    aFcnTruthTableAction_5();
end

function aFcnTruthTableAction_1()

% happy

e=7;

function aFcnTruthTableAction_2()

% excited

e=8;

function aFcnTruthTableAction_3()

% fear

e=4;

function aFcnTruthTableAction_4()

% frustration

e=3;

function aFcnTruthTableAction_5()

% pleased

e=6;

function aFcnTruthTableAction_6()

% contempt

e=5;

function aFcnTruthTableAction_7()

% bored

e=1;

function aFcnTruthTableAction_8()

% sad

e=2;

== matlab function Demo_AUV_VA/EmotionGeneration/calculateValenceArousal/HELN_VA_Emo ==
  data: V input; e output double size=1; A input double
function e = fcn(V, A)

aVarTruthTableCondition_1 = false;
aVarTruthTableCondition_2 = false;
aVarTruthTableCondition_3 = false;
aVarTruthTableCondition_4 = false;
aVarTruthTableCondition_5 = false;
aVarTruthTableCondition_6 = false;
aVarTruthTableCondition_7 = false;
aVarTruthTableCondition_8 = false;


% 7-happy  2,1

aVarTruthTableCondition_1 = logical(V>10 && A<40 && A>10);

% 8-ex  1,2 AND 2,2

aVarTruthTableCondition_2 = logical(V>0 && A>40);

% 4-fear  -1,2 AND -2,2

aVarTruthTableCondition_3 = logical(V<0 && A>40);

% 3-frust  -2,1

aVarTruthTableCondition_4 = logical(V<-10 && A<40 && A>10);

% 6-idle  2,-1

aVarTruthTableCondition_5 = logical(V>10 && A<-10 && A>-40);

% 5-calm  1,-2 AND 2,-2

aVarTruthTableCondition_6 = logical(V>0 && A<-40);

% 1-bored  -1,-2 AND -2,-2

aVarTruthTableCondition_7 = logical(V<0 && A<-40);

% 2-sad  -2,-1

aVarTruthTableCondition_8 = logical(V<-10 && A<-10 && A>-40);

if (aVarTruthTableCondition_1)
    aFcnTruthTableAction_1();
elseif (aVarTruthTableCondition_2)
    aFcnTruthTableAction_2();
elseif (aVarTruthTableCondition_3)
    aFcnTruthTableAction_3();
elseif (aVarTruthTableCondition_4)
    aFcnTruthTableAction_4();
elseif (aVarTruthTableCondition_5)
    aFcnTruthTableAction_5();
elseif (aVarTruthTableCondition_6)
    aFcnTruthTableAction_6();
elseif (aVarTruthTableCondition_7)
    aFcnTruthTableAction_7();
elseif (aVarTruthTableCondition_8)
    aFcnTruthTableAction_8();
else % Default
    aFcnTruthTableAction_5();
end

function aFcnTruthTableAction_1()

% happy

e=7;

function aFcnTruthTableAction_2()

% excited

e=8;

function aFcnTruthTableAction_3()

% fear

e=4;

function aFcnTruthTableAction_4()

% frustration

e=3;

function aFcnTruthTableAction_5()

% idle

e=6;

function aFcnTruthTableAction_6()

% contempt

e=5;

function aFcnTruthTableAction_7()

% bored

e=1;

function aFcnTruthTableAction_8()

% sad

e=2;

== matlab function Demo_AUV_VA/EmotionGeneration/calculateValenceArousal/LELN_VA_Emo ==
  data: V input; e output double size=1; A input double
function e = fcn(V, A)

aVarTruthTableCondition_1 = false;
aVarTruthTableCondition_2 = false;
aVarTruthTableCondition_3 = false;
aVarTruthTableCondition_4 = false;
aVarTruthTableCondition_5 = false;
aVarTruthTableCondition_6 = false;
aVarTruthTableCondition_7 = false;
aVarTruthTableCondition_8 = false;


% 7-happy  2,1

aVarTruthTableCondition_1 = logical(V>20 && A<40 && A>20);

% 8-ex  1,2 AND 2,2

aVarTruthTableCondition_2 = logical(V>0 && A>40);

% 4-fear  -1,2 AND -2,2

aVarTruthTableCondition_3 = logical(V<0 && A>40);

% 3-frust  -2,1

aVarTruthTableCondition_4 = logical(V<-20 && A<40 && A>20);

% 6-idle  2,-1

aVarTruthTableCondition_5 = logical(V>20 && A<-20 && A>-40);

% 5-calm  1,-2 AND 2,-2

aVarTruthTableCondition_6 = logical(V>0 && A<-40);

% 1-bored  -1,-2 AND -2,-2

aVarTruthTableCondition_7 = logical(V<0 && A<-40);

% 2-sad  -2,-1

aVarTruthTableCondition_8 = logical(V<-20 && A<-20 && A>-40);

if (aVarTruthTableCondition_1)
    aFcnTruthTableAction_1();
elseif (aVarTruthTableCondition_2)
    aFcnTruthTableAction_2();
elseif (aVarTruthTableCondition_3)
    aFcnTruthTableAction_3();
elseif (aVarTruthTableCondition_4)
    aFcnTruthTableAction_4();
elseif (aVarTruthTableCondition_5)
    aFcnTruthTableAction_5();
elseif (aVarTruthTableCondition_6)
    aFcnTruthTableAction_6();
elseif (aVarTruthTableCondition_7)
    aFcnTruthTableAction_7();
elseif (aVarTruthTableCondition_8)
    aFcnTruthTableAction_8();
else % Default
    aFcnTruthTableAction_5();
end

function aFcnTruthTableAction_1()

% happy

e=7;

function aFcnTruthTableAction_2()

% excited

e=8;

function aFcnTruthTableAction_3()

% fear

e=4;

function aFcnTruthTableAction_4()

% frustration

e=3;

function aFcnTruthTableAction_5()

% idle

e=6;

function aFcnTruthTableAction_6()

% contempt

e=5;

function aFcnTruthTableAction_7()

% bored

e=1;

function aFcnTruthTableAction_8()

% sad

e=2;

== matlab function Demo_AUV_VA/EmotionGeneration/calculateValenceArousal/HEHN plot ==
  data: v input; a input
function fcn(v,a)
%coder.extrinsic to bypass code generation
coder.extrinsic('fscanf')
coder.extrinsic('get_param');
% coder.extrinsic('importdata');

currentTime=get_param('Demo_EP_IdleRandMerg','SimulationTime');%use name of simulink proj

A = [v;a;currentTime];
fileID = fopen('HEHN_VA_table.txt','a');
fprintf(fileID,'%0.1f,%0.1f,%0.1f\r\n',A);
fclose(fileID);

% matrix = importdata('HEHN_VA_table.txt',','); 
% tri = delaunay(matrix(:,1),matrix(:,2));
% trisurf(tri,matrix(:,1),matrix(:,2),matrix(:,3))
% shading interp
% colorbar

%-----------------------------------------
% fileID = fopen('HEHN_VA_table.txt','r');
% formatSpec = '%1f\r %1f\r %1f\r\n';
% sizeA = [3 Inf];
% A = fscanf(fileID,formatSpec,sizeA)
% % A = A'
% fclose(fileID);

% x = zeros(100,2);y = zeros(100,2);
% filename = 'HEHN_VA_table.txt';
% delimiterIn = ' ';
% headerlinesIn = 1;
% A = importdata(filename,delimiterIn,headerlinesIn);

% fileID=fopen('HEHN_VA_table4.txt');
% s=textscan(fileID,'%d %d %d','headerlines',23);
% fclose(fileID);
% x=s{1}

== matlab function Demo_AUV_VA/EmotionGeneration/calculateValenceArousal/LEHN plot ==
  data: v input; a input
function fcn(v,a)
%coder.extrinsic to bypass code generation
coder.extrinsic('fscanf')
coder.extrinsic('get_param');
% coder.extrinsic('importdata');

currentTime=get_param('Demo_EP_IdleRandMerg','SimulationTime');%use name of simulink proj

A = [v;a;currentTime];

fileID = fopen('LEHN_VA_table.txt','a');
fprintf(fileID,'%0.1f,%0.1f,%0.1f\r\n',A);
fclose(fileID);

%use the following to draw the plot
%tmp_data = importdata('HEHN_VA_table.txt',','); 
%no need: x=tmp_data(:,1);y=tmp_data(:,2);z=tmp_data(:,3)
%matrix=tmp_data
%tri = delaunay(matrix(:,1),matrix(:,2));
%trisurf(tri,matrix(:,1),matrix(:,2),matrix(:,3))
%shading interp

%-----------------------------------------
% fileID = fopen('HEHN_VA_table.txt','r');
% formatSpec = '%1f\r %1f\r %1f\r\n';
% sizeA = [3 Inf];
% A = fscanf(fileID,formatSpec,sizeA)
% % A = A'
% fclose(fileID);

% x = zeros(100,2);y = zeros(100,2);
% filename = 'HEHN_VA_table.txt';
% delimiterIn = ' ';
% headerlinesIn = 1;
% A = importdata(filename,delimiterIn,headerlinesIn);

% fileID=fopen('HEHN_VA_table4.txt');
% s=textscan(fileID,'%d %d %d','headerlines',23);
% fclose(fileID);
% x=s{1}

== matlab function Demo_AUV_VA/EmotionGeneration/calculateValenceArousal/HELN plot ==
  data: v input; a input
function fcn(v,a)
%coder.extrinsic to bypass code generation
coder.extrinsic('fscanf')
coder.extrinsic('get_param');
% coder.extrinsic('importdata');

currentTime=get_param('Demo_EP_IdleRandMerg','SimulationTime');%use name of simulink proj

A = [v;a;currentTime];

fileID = fopen('HELN_VA_table.txt','a');
fprintf(fileID,'%0.1f,%0.1f,%0.1f\r\n',A);
fclose(fileID);

%use the following to draw the plot
%tmp_data = importdata('HEHN_VA_table.txt',','); 
%no need: x=tmp_data(:,1);y=tmp_data(:,2);z=tmp_data(:,3)
%matrix=tmp_data
%tri = delaunay(matrix(:,1),matrix(:,2));
%trisurf(tri,matrix(:,1),matrix(:,2),matrix(:,3))
%shading interp

%-----------------------------------------
% fileID = fopen('HEHN_VA_table.txt','r');
% formatSpec = '%1f\r %1f\r %1f\r\n';
% sizeA = [3 Inf];
% A = fscanf(fileID,formatSpec,sizeA)
% % A = A'
% fclose(fileID);

% x = zeros(100,2);y = zeros(100,2);
% filename = 'HEHN_VA_table.txt';
% delimiterIn = ' ';
% headerlinesIn = 1;
% A = importdata(filename,delimiterIn,headerlinesIn);

% fileID=fopen('HEHN_VA_table4.txt');
% s=textscan(fileID,'%d %d %d','headerlines',23);
% fclose(fileID);
% x=s{1}

== matlab function Demo_AUV_VA/EmotionGeneration/calculateValenceArousal/LELN plot ==
  data: v input; a input
function fcn(v,a)
%coder.extrinsic to bypass code generation
coder.extrinsic('fscanf')
coder.extrinsic('get_param');
% coder.extrinsic('importdata');

currentTime=get_param('Demo_EP_IdleRandMerg','SimulationTime');%use name of simulink proj

A = [v;a;currentTime];

fileID = fopen('LELN_VA_table.txt','a');
fprintf(fileID,'%0.1f,%0.1f,%0.1f\r\n',A);
fclose(fileID);

%use the following to draw the plot
%matrix = importdata('HEHN_VA_table.txt',','); 
%tri = delaunay(matrix(:,1),matrix(:,2));
%trisurf(tri,matrix(:,1),matrix(:,2),matrix(:,3))
%shading interp
%colorbar
%-----------------------------------------
% fileID = fopen('HEHN_VA_table.txt','r');
% formatSpec = '%1f\r %1f\r %1f\r\n';
% sizeA = [3 Inf];
% A = fscanf(fileID,formatSpec,sizeA)
% % A = A'
% fclose(fileID);

% x = zeros(100,2);y = zeros(100,2);
% filename = 'HEHN_VA_table.txt';
% delimiterIn = ' ';
% headerlinesIn = 1;
% A = importdata(filename,delimiterIn,headerlinesIn);

% fileID=fopen('HEHN_VA_table4.txt');
% s=textscan(fileID,'%d %d %d','headerlines',23);
% fclose(fileID);
% x=s{1}
